simulink model "GTA_PCMFirmware"  (Simulink 7.8)
settings: Solver=FixedStepDiscrete  StartTime=0.0  StopTime=10.0  RelTol=1e-3
PreLoadFcn:
  | try, eval([bdroot '_setup']); catch, eval('model_setup', ''); end
InitFcn:
  | try, eval([bdroot '_setup']); catch, eval('model_setup', ''); end
undefined symbols (not defined in the file): fndFwd, fndNeut, fndRev, FWDlockout, GCM, keySwIgn2, motohawk_build_version, motohawk_trunc_name, motohawk_vardec_path, REVlockout
libraries: MotoHawk_lib x313, simulink x47, GTA_Library x13
(part 3 of 7)

== system GTA_PCMFirmware/Function/1 Inputs and Paramaters/Limits/Pb ==
  Mux : Mux  Inputs=13
  motohawk_calibration : MotoHawk_lib/Calibration & Probing Blocks/motohawk_calibration  nam='PbMaxCellVoltage'  val=PbMaxCellVoltage  storage=Calibration  show_more=off  name_source=Use Parameter  data_type=Inherit from 'Default Value'  read_level=1  write_level=1  ovr_cals=on  view_as=Number  enum_struct={'Disabled', 'Enabled'}  vector_style=Wide Row  use_help_units=off  help=''  units=''  use_header_enum=off  row_header_enum={}  col_header_enum={}  use_min_max=off  min_val=-inf  max_val=inf  use_precision=off  precision=''  gain=1  offset=0  exp=1  use_mototune_group=off  mototune_group=motohawk_vardec_path(gcb)
  motohawk_calibration1 : MotoHawk_lib/Calibration & Probing Blocks/motohawk_calibration  nam='PbMinCellVoltage'  val=PbMinCellVoltage  storage=Calibration  show_more=off  name_source=Use Parameter  data_type=Inherit from 'Default Value'  read_level=1  write_level=1  ovr_cals=on  view_as=Number  enum_struct={'Disabled', 'Enabled'}  vector_style=Wide Row  use_help_units=off  help=''  units=''  use_header_enum=off  row_header_enum={}  col_header_enum={}  use_min_max=off  min_val=-inf  max_val=inf  use_precision=off  precision=''  gain=1  offset=0  exp=1  use_mototune_group=off  mototune_group=motohawk_vardec_path(gcb)
  motohawk_calibration10 : MotoHawk_lib/Calibration & Probing Blocks/motohawk_calibration  nam='PbMotorCurrentScalar'  val=PbMotorCurrentScalar  storage=Calibration  show_more=off  name_source=Use Parameter  data_type=Inherit from 'Default Value'  read_level=1  write_level=1  ovr_cals=on  view_as=Number  enum_struct={'Disabled', 'Enabled'}  vector_style=Wide Row  use_help_units=off  help=''  units=''  use_header_enum=off  row_header_enum={}  col_header_enum={}  use_min_max=off  min_val=-inf  max_val=inf  use_precision=off  precision=''  gain=1  offset=0  exp=1  use_mototune_group=off  mototune_group=motohawk_vardec_path(gcb)
  motohawk_calibration11 : MotoHawk_lib/Calibration & Probing Blocks/motohawk_calibration  nam='PbMotorRegenScalar'  val=PbMotorRegenScalar  storage=Calibration  show_more=off  name_source=Use Parameter  data_type=Inherit from 'Default Value'  read_level=1  write_level=1  ovr_cals=on  view_as=Number  enum_struct={'Disabled', 'Enabled'}  vector_style=Wide Row  use_help_units=off  help=''  units=''  use_header_enum=off  row_header_enum={}  col_header_enum={}  use_min_max=off  min_val=-inf  max_val=inf  use_precision=off  precision=''  gain=1  offset=0  exp=1  use_mototune_group=off  mototune_group=motohawk_vardec_path(gcb)
  motohawk_calibration12 : MotoHawk_lib/Calibration & Probing Blocks/motohawk_calibration  nam='PbMaxRegenVoltage'  val=PbMaxRegenVoltage  storage=Calibration  show_more=off  name_source=Use Parameter  data_type=Inherit from 'Default Value'  read_level=1  write_level=1  ovr_cals=on  view_as=Number  enum_struct={'Disabled', 'Enabled'}  vector_style=Wide Row  use_help_units=off  help=''  units=''  use_header_enum=off  row_header_enum={}  col_header_enum={}  use_min_max=off  min_val=-inf  max_val=inf  use_precision=off  precision=''  gain=1  offset=0  exp=1  use_mototune_group=off  mototune_group=motohawk_vardec_path(gcb)
  motohawk_calibration2 : MotoHawk_lib/Calibration & Probing Blocks/motohawk_calibration  nam='PbCurrentLimit'  val=PbCurrentLimit  storage=Calibration  show_more=off  name_source=Use Parameter  data_type=Inherit from 'Default Value'  read_level=1  write_level=1  ovr_cals=on  view_as=Number  enum_struct={'Disabled', 'Enabled'}  vector_style=Wide Row  use_help_units=off  help=''  units=''  use_header_enum=off  row_header_enum={}  col_header_enum={}  use_min_max=off  min_val=-inf  max_val=inf  use_precision=off  precision=''  gain=1  offset=0  exp=1  use_mototune_group=off  mototune_group=motohawk_vardec_path(gcb)
  motohawk_calibration3 : MotoHawk_lib/Calibration & Probing Blocks/motohawk_calibration  nam='PbRegenLimit'  val=PbRegenLimit  storage=Calibration  show_more=off  name_source=Use Parameter  data_type=Inherit from 'Default Value'  read_level=1  write_level=1  ovr_cals=on  view_as=Number  enum_struct={'Disabled', 'Enabled'}  vector_style=Wide Row  use_help_units=off  help=''  units=''  use_header_enum=off  row_header_enum={}  col_header_enum={}  use_min_max=off  min_val=-inf  max_val=inf  use_precision=off  precision=''  gain=1  offset=0  exp=1  use_mototune_group=off  mototune_group=motohawk_vardec_path(gcb)
  motohawk_calibration4 : MotoHawk_lib/Calibration & Probing Blocks/motohawk_calibration  nam='PbMaxChargeTemp'  val=PbMaxChargeTemp  storage=Calibration  show_more=off  name_source=Use Parameter  data_type=Inherit from 'Default Value'  read_level=1  write_level=1  ovr_cals=on  view_as=Number  enum_struct={'Disabled', 'Enabled'}  vector_style=Wide Row  use_help_units=off  help=''  units=''  use_header_enum=off  row_header_enum={}  col_header_enum={}  use_min_max=off  min_val=-inf  max_val=inf  use_precision=off  precision=''  gain=1  offset=0  exp=1  use_mototune_group=off  mototune_group=motohawk_vardec_path(gcb)
  motohawk_calibration5 : MotoHawk_lib/Calibration & Probing Blocks/motohawk_calibration  nam='PbMinChargeTemp'  val=PbMinChargeTemp  storage=Calibration  show_more=off  name_source=Use Parameter  data_type=Inherit from 'Default Value'  read_level=1  write_level=1  ovr_cals=on  view_as=Number  enum_struct={'Disabled', 'Enabled'}  vector_style=Wide Row  use_help_units=off  help=''  units=''  use_header_enum=off  row_header_enum={}  col_header_enum={}  use_min_max=off  min_val=-inf  max_val=inf  use_precision=off  precision=''  gain=1  offset=0  exp=1  use_mototune_group=off  mototune_group=motohawk_vardec_path(gcb)
  motohawk_calibration6 : MotoHawk_lib/Calibration & Probing Blocks/motohawk_calibration  nam='PbMaxDischargeTemp'  val=PbMaxDischargeTemp  storage=Calibration  show_more=off  name_source=Use Parameter  data_type=Inherit from 'Default Value'  read_level=1  write_level=1  ovr_cals=on  view_as=Number  enum_struct={'Disabled', 'Enabled'}  vector_style=Wide Row  use_help_units=off  help=''  units=''  use_header_enum=off  row_header_enum={}  col_header_enum={}  use_min_max=off  min_val=-inf  max_val=inf  use_precision=off  precision=''  gain=1  offset=0  exp=1  use_mototune_group=off  mototune_group=motohawk_vardec_path(gcb)
  motohawk_calibration7 : MotoHawk_lib/Calibration & Probing Blocks/motohawk_calibration  nam='PbMinDischargeTemp'  val=PbMinDischargeTemp  storage=Calibration  show_more=off  name_source=Use Parameter  data_type=Inherit from 'Default Value'  read_level=1  write_level=1  ovr_cals=on  view_as=Number  enum_struct={'Disabled', 'Enabled'}  vector_style=Wide Row  use_help_units=off  help=''  units=''  use_header_enum=off  row_header_enum={}  col_header_enum={}  use_min_max=off  min_val=-inf  max_val=inf  use_precision=off  precision=''  gain=1  offset=0  exp=1  use_mototune_group=off  mototune_group=motohawk_vardec_path(gcb)
  motohawk_calibration8 : MotoHawk_lib/Calibration & Probing Blocks/motohawk_calibration  nam='PbMaxPackVoltage'  val=PbMaxPackVoltage  storage=Calibration  show_more=off  name_source=Use Parameter  data_type=Inherit from 'Default Value'  read_level=1  write_level=1  ovr_cals=on  view_as=Number  enum_struct={'Disabled', 'Enabled'}  vector_style=Wide Row  use_help_units=off  help=''  units=''  use_header_enum=off  row_header_enum={}  col_header_enum={}  use_min_max=off  min_val=-inf  max_val=inf  use_precision=off  precision=''  gain=1  offset=0  exp=1  use_mototune_group=off  mototune_group=motohawk_vardec_path(gcb)
  motohawk_calibration9 : MotoHawk_lib/Calibration & Probing Blocks/motohawk_calibration  nam='PbMinPackVoltage'  val=PbMinPackVoltage  storage=Calibration  show_more=off  name_source=Use Parameter  data_type=Inherit from 'Default Value'  read_level=1  write_level=1  ovr_cals=on  view_as=Number  enum_struct={'Disabled', 'Enabled'}  vector_style=Wide Row  use_help_units=off  help=''  units=''  use_header_enum=off  row_header_enum={}  col_header_enum={}  use_min_max=off  min_val=-inf  max_val=inf  use_precision=off  precision=''  gain=1  offset=0  exp=1  use_mototune_group=off  mototune_group=motohawk_vardec_path(gcb)
  PbPack : Outport
  wires:
  Mux/1 -> PbPack/1
  motohawk_calibration12/1 -> Mux/13  "MaxRegenVoltage"
  motohawk_calibration11/1 -> Mux/12  "MotorRegenScalar"
  motohawk_calibration10/1 -> Mux/11  "MotorCurrentScalar"
  motohawk_calibration9/1 -> Mux/10  "MinPackVoltage"
  motohawk_calibration8/1 -> Mux/9  "MaxPackVoltage"
  motohawk_calibration7/1 -> Mux/8  "MinDischargeTemp"
  motohawk_calibration6/1 -> Mux/7  "MaxDischargeTemp"
  motohawk_calibration5/1 -> Mux/6  "MinChargeTemp"
  motohawk_calibration4/1 -> Mux/5  "MaxChargeTemp"
  motohawk_calibration3/1 -> Mux/4  "RegenLimit"
  motohawk_calibration2/1 -> Mux/3  "CurrentLimit"
  motohawk_calibration1/1 -> Mux/2  "MinCellVoltage"
  motohawk_calibration/1 -> Mux/1  "MaxCellVoltage"

== system GTA_PCMFirmware/Function/2 Control Loop/Component Controls/Body Control ==
  SYSin : Inport
  MotorControl : Inport  Port=2
  Bus Creator : BusCreator  Inputs=3
  Defroster : Subsystem
  Inter Wiper : Subsystem
  Reverse Lights : Subsystem
  Out : Outport
  wires:
  SYSin/1 -> Defroster/1(SYSin), Inter Wiper/1(SYSin), Reverse Lights/1(SYSin)
  Inter Wiper/1(Out1) -> Bus Creator/2  "Wiper"
  Defroster/1(Out1) -> Bus Creator/1  "Defrost"
  Reverse Lights/1(Out1) -> Bus Creator/3  "ReverseLight"
  Bus Creator/1 -> Out/1
  MotorControl/1 -> Reverse Lights/2(MotorControl)

== system GTA_PCMFirmware/Function/2 Control Loop/Component Controls/Charger Control ==
  SYSin : Inport
  Bus Creator : BusCreator  Inputs=1
  Bus Selector : BusSelector  OutputSignals=ModeControl.ChargeEnable,BUS.Input Bus.CANin.BMS.csChargeFlags.PackCharging
  Logical Operator : Logic  AllPortsSameDT=off  OutDataTypeStr=boolean
  Out : Outport
  wires:
  SYSin/1 -> Bus Selector/1
  Bus Selector/1 -> Logical Operator/1  "<ChargeEnable>"
  Bus Selector/2 -> Logical Operator/2  "<PackCharging>"
  Logical Operator/1 -> Bus Creator/1  "ChargerOut"
  Bus Creator/1 -> Out/1

== system GTA_PCMFirmware/Function/2 Control Loop/Component Controls/Display Control ==
  SYSin : Inport
  MotorControl : Inport  Port=2
  Bus Creator : BusCreator
  Fault Lamps : Subsystem
  Gearbox Display : Subsystem
  ReadyLight : Subsystem
  Vehicle Speed : Subsystem
  Out : Outport
  wires:
  SYSin/1 -> Fault Lamps/1(SYSin), Gearbox Display/1(SYSin), Vehicle Speed/1(SYSin), ReadyLight/1(SYSin)
  Fault Lamps/1(FaultLights) -> Bus Creator/1  "FaultLamp"
  Vehicle Speed/1(Out1) -> Bus Creator/3  "VehSpeed"
  Gearbox Display/1(GboxPos) -> Bus Creator/2  "GearDisp"
  Bus Creator/1 -> Out/1
  ReadyLight/1(ReadyLight) -> Bus Creator/4  "ReadyLight"
  MotorControl/1 -> Gearbox Display/2(MotorControl)

== system GTA_PCMFirmware/Function/2 Control Loop/Component Controls/Motor Control ==
  SYSin : Inport
  Bus Creator : BusCreator  Inputs=3
  Bus Selector : BusSelector  OutputSignals=ModeControl.DriveEnable,BUS.Input Bus.CANin.Motor Controller.KinVoltSpeed.ErrorField
  Bus Selector1 : BusSelector  OutputSignals=BUS.Input Bus.DigitalIn.Shifter.ShifterPos,BUS.Input Bus.CANin.Motor Controller.KinVoltSpeed.MotorSpeed,BUS.Input Bus.CANin.Motor Controller.KinCurrFB.iq_ref
  Bus Selector2 : BusSelector  OutputSignals=ModeControl.MotorEnable,BUS.Input Bus.DigitalIn.Shifter.ShifterPos,BUS.Input Bus.DigitalIn.KeySwitch.KeySw,BUS.Input Bus.AnalogIn.ThrottlePedal.PedalPerc,BUS.Input Bus.CANin.Motor Controller.KinVoltSpeed.MotorSpeed,BUS.Current Limit.TorqueLimit.MaxCurrPerc,BUS.Current Limit.RegenLimit.MaxRegenPerc,BUS.Input Bus.Limits.BattLimits.MotorRegenScalar,BUS.Input Bus.Limits.BattLimits.MotorCurrentScalar
  Current Request Algorithm : Subsystem
  Direction Lockout : Subsystem
  Direction Selector & Control Loop : Subsystem
  Enable : Subsystem
  Out : Outport
  wires:
  Enable/1(enable) -> Bus Creator/1
  Direction Lockout/1(" FNDOut") -> Direction Selector & Control Loop/1(" FNDSw"), Current Request Algorithm/4(FNDOut), Bus Creator/2
  Bus Selector1/1 -> Direction Lockout/1(" FNDSw")  "<ShifterPos>"
  Bus Selector1/2 -> Direction Selector & Control Loop/4(Speed), Direction Lockout/2(" Speed")  "<MotorSpeed>"
  Current Request Algorithm/1(torqueRequest) -> Direction Selector & Control Loop/2(" torque")
  Direction Selector & Control Loop/1(torqueOutput) -> Bus Creator/3
  Bus Selector1/3 -> Direction Selector & Control Loop/3(CurFBK)  "<iq_ref>"
  Bus Selector/1 -> Enable/1("driveEnable ")  "<DriveEnable>"
  Bus Selector/2 -> Enable/2(errorField)  "<ErrorField>"
  SYSin/1 -> Bus Selector1/1, Bus Selector/1, Bus Selector2/1
  Bus Selector2/1 -> Current Request Algorithm/1(MotorEnable)  "<MotorEnable>"
  Bus Selector2/2 -> Current Request Algorithm/2("FNDSwitch ")  "<ShifterPos>"
  Bus Selector2/3 -> Current Request Algorithm/3(KeySwitch)  "<KeySw>"
  Bus Selector2/4 -> Current Request Algorithm/5("Pedal ")  "<PedalPerc>"
  Bus Selector2/5 -> Current Request Algorithm/6(Speed)  "<MotorSpeed>"
  Bus Selector2/6 -> Current Request Algorithm/7("TorqueLim ")  "<MaxCurrPerc>"
  Bus Selector2/7 -> Current Request Algorithm/8(RegenLim)  "<MaxRegenPerc>"
  Bus Selector2/8 -> Current Request Algorithm/9(RegenScalar)  "<MotorRegenScalar>"
  Bus Selector2/9 -> Current Request Algorithm/10(CurrentScalar)  "<MotorCurrentScalar>"
  Bus Creator/1 -> Out/1

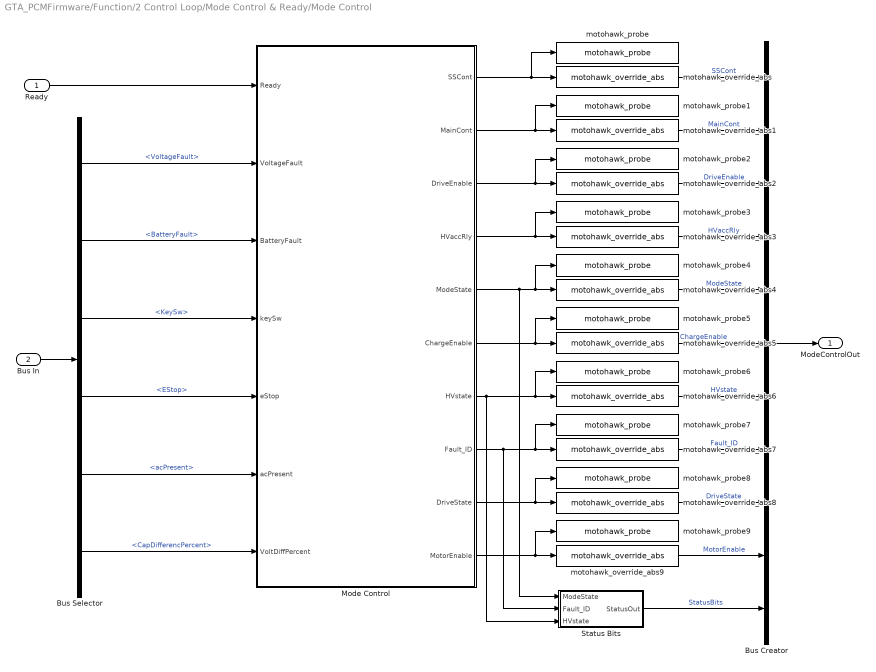
== system GTA_PCMFirmware/Function/2 Control Loop/Mode Control & Ready/Mode Control ==
  Ready : Inport
  Bus In : Inport  Port=2
  Bus Creator : BusCreator  Inputs=11
  Bus Selector : BusSelector  OutputSignals=Voltage level.VoltageFault,Faults.BatteryFault.BatteryFault,Input Bus.DigitalIn.KeySwitch.KeySw,Input Bus.DigitalIn.EStop.EStop,Input Bus.DigitalIn.Charger.acPresent,Voltage level.CapDifferencPercent
  Mode Control : Stateflow chart  TreatAsAtomicUnit=on
  Status Bits : Subsystem
  motohawk_override_abs : MotoHawk_lib/Calibration & Probing Blocks/motohawk_override_abs  parent_name='SScont'  parent_val=0  show_more=off  name_source=Use Parameter  parent_read_level=1  parent_override_level=1  view_as=Number  enum_struct={'Disabled', 'Enabled'}  use_help_units=off  parent_help=''  parent_units=''  use_min_max=off  parent_min=-inf  parent_max=inf  use_precision=off  parent_precision=''  parent_gain=1  parent_offset=0  parent_exp=1  use_mototune_group=off  parent_group=motohawk_vardec_path(gcb)
  motohawk_override_abs1 : MotoHawk_lib/Calibration & Probing Blocks/motohawk_override_abs  parent_name='MainCont'  parent_val=0  show_more=off  name_source=Use Parameter  parent_read_level=1  parent_override_level=1  view_as=Number  enum_struct={'Disabled', 'Enabled'}  use_help_units=off  parent_help=''  parent_units=''  use_min_max=off  parent_min=-inf  parent_max=inf  use_precision=off  parent_precision=''  parent_gain=1  parent_offset=0  parent_exp=1  use_mototune_group=off  parent_group=motohawk_vardec_path(gcb)
  motohawk_override_abs2 : MotoHawk_lib/Calibration & Probing Blocks/motohawk_override_abs  parent_name='DriveEnable'  parent_val=0  show_more=off  name_source=Use Parameter  parent_read_level=1  parent_override_level=1  view_as=Number  enum_struct={'Disabled', 'Enabled'}  use_help_units=off  parent_help=''  parent_units=''  use_min_max=off  parent_min=-inf  parent_max=inf  use_precision=off  parent_precision=''  parent_gain=1  parent_offset=0  parent_exp=1  use_mototune_group=off  parent_group=motohawk_vardec_path(gcb)
  motohawk_override_abs3 : MotoHawk_lib/Calibration & Probing Blocks/motohawk_override_abs  parent_name='HVaccRly'  parent_val=0  show_more=off  name_source=Use Parameter  parent_read_level=1  parent_override_level=1  view_as=Number  enum_struct={'Disabled', 'Enabled'}  use_help_units=off  parent_help=''  parent_units=''  use_min_max=off  parent_min=-inf  parent_max=inf  use_precision=off  parent_precision=''  parent_gain=1  parent_offset=0  parent_exp=1  use_mototune_group=off  parent_group=motohawk_vardec_path(gcb)
  motohawk_override_abs4 : MotoHawk_lib/Calibration & Probing Blocks/motohawk_override_abs  parent_name='ModeState'  parent_val=0  show_more=off  name_source=Use Parameter  parent_read_level=1  parent_override_level=1  view_as=Number  enum_struct={'Disabled', 'Enabled'}  use_help_units=off  parent_help=''  parent_units=''  use_min_max=off  parent_min=-inf  parent_max=inf  use_precision=off  parent_precision=''  parent_gain=1  parent_offset=0  parent_exp=1  use_mototune_group=off  parent_group=motohawk_vardec_path(gcb)
  motohawk_override_abs5 : MotoHawk_lib/Calibration & Probing Blocks/motohawk_override_abs  parent_name='ChargeEnable'  parent_val=0  show_more=off  name_source=Use Parameter  parent_read_level=1  parent_override_level=1  view_as=Number  enum_struct={'Disabled', 'Enabled'}  use_help_units=off  parent_help=''  parent_units=''  use_min_max=off  parent_min=-inf  parent_max=inf  use_precision=off  parent_precision=''  parent_gain=1  parent_offset=0  parent_exp=1  use_mototune_group=off  parent_group=motohawk_vardec_path(gcb)
  motohawk_override_abs6 : MotoHawk_lib/Calibration & Probing Blocks/motohawk_override_abs  parent_name='HVstate'  parent_val=0  show_more=off  name_source=Use Parameter  parent_read_level=1  parent_override_level=1  view_as=Number  enum_struct={'Disabled', 'Enabled'}  use_help_units=off  parent_help=''  parent_units=''  use_min_max=off  parent_min=-inf  parent_max=inf  use_precision=off  parent_precision=''  parent_gain=1  parent_offset=0  parent_exp=1  use_mototune_group=off  parent_group=motohawk_vardec_path(gcb)
  motohawk_override_abs7 : MotoHawk_lib/Calibration & Probing Blocks/motohawk_override_abs  parent_name='Fault_ID'  parent_val=0  show_more=off  name_source=Use Parameter  parent_read_level=1  parent_override_level=1  view_as=Number  enum_struct={'Disabled', 'Enabled'}  use_help_units=off  parent_help=''  parent_units=''  use_min_max=off  parent_min=-inf  parent_max=inf  use_precision=off  parent_precision=''  parent_gain=1  parent_offset=0  parent_exp=1  use_mototune_group=off  parent_group=motohawk_vardec_path(gcb)
  motohawk_override_abs8 : MotoHawk_lib/Calibration & Probing Blocks/motohawk_override_abs  parent_name='DriveState'  parent_val=0  show_more=off  name_source=Use Parameter  parent_read_level=1  parent_override_level=1  view_as=Number  enum_struct={'Disabled', 'Enabled'}  use_help_units=off  parent_help=''  parent_units=''  use_min_max=off  parent_min=-inf  parent_max=inf  use_precision=off  parent_precision=''  parent_gain=1  parent_offset=0  parent_exp=1  use_mototune_group=off  parent_group=motohawk_vardec_path(gcb)
  motohawk_override_abs9 : MotoHawk_lib/Calibration & Probing Blocks/motohawk_override_abs  parent_name='MotorEnable'  parent_val=0  show_more=off  name_source=Use Parameter  parent_read_level=1  parent_override_level=1  view_as=Number  enum_struct={'Disabled', 'Enabled'}  use_help_units=off  parent_help=''  parent_units=''  use_min_max=off  parent_min=-inf  parent_max=inf  use_precision=off  parent_precision=''  parent_gain=1  parent_offset=0  parent_exp=1  use_mototune_group=off  parent_group=motohawk_vardec_path(gcb)
  motohawk_probe : MotoHawk_lib/Calibration & Probing Blocks/motohawk_probe  nam='SScont'  show_more=off  name_source=Use Parameter  read_level=1  view_as=Number  enum_struct={'Disabled', 'Enabled'}  vector_style=Wide Row  use_help_units=off  help=''  units=''  use_header_enum=off  row_header_enum={}  col_header_enum={}  use_min_max=off  min_val=-inf  max_val=inf  use_precision=off  precision=''  gain=1  offset=0  exp=1  use_mototune_group=off  mototune_group=motohawk_vardec_path(gcb)
  motohawk_probe1 : MotoHawk_lib/Calibration & Probing Blocks/motohawk_probe  nam='MainCont'  show_more=off  name_source=Use Parameter  read_level=1  view_as=Number  enum_struct={'Disabled', 'Enabled'}  vector_style=Wide Row  use_help_units=off  help=''  units=''  use_header_enum=off  row_header_enum={}  col_header_enum={}  use_min_max=off  min_val=-inf  max_val=inf  use_precision=off  precision=''  gain=1  offset=0  exp=1  use_mototune_group=off  mototune_group=motohawk_vardec_path(gcb)
  motohawk_probe2 : MotoHawk_lib/Calibration & Probing Blocks/motohawk_probe  nam='DriveEnable'  show_more=off  name_source=Use Parameter  read_level=1  view_as=Number  enum_struct={'Disabled', 'Enabled'}  vector_style=Wide Row  use_help_units=off  help=''  units=''  use_header_enum=off  row_header_enum={}  col_header_enum={}  use_min_max=off  min_val=-inf  max_val=inf  use_precision=off  precision=''  gain=1  offset=0  exp=1  use_mototune_group=off  mototune_group=motohawk_vardec_path(gcb)
  motohawk_probe3 : MotoHawk_lib/Calibration & Probing Blocks/motohawk_probe  nam='HVaccRly'  show_more=off  name_source=Use Parameter  read_level=1  view_as=Number  enum_struct={'Disabled', 'Enabled'}  vector_style=Wide Row  use_help_units=off  help=''  units=''  use_header_enum=off  row_header_enum={}  col_header_enum={}  use_min_max=off  min_val=-inf  max_val=inf  use_precision=off  precision=''  gain=1  offset=0  exp=1  use_mototune_group=off  mototune_group=motohawk_vardec_path(gcb)
  motohawk_probe4 : MotoHawk_lib/Calibration & Probing Blocks/motohawk_probe  nam='ModeState'  show_more=off  name_source=Use Parameter  read_level=1  view_as=Number  enum_struct={'Disabled', 'Enabled'}  vector_style=Wide Row  use_help_units=off  help=''  units=''  use_header_enum=off  row_header_enum={}  col_header_enum={}  use_min_max=off  min_val=-inf  max_val=inf  use_precision=off  precision=''  gain=1  offset=0  exp=1  use_mototune_group=off  mototune_group=motohawk_vardec_path(gcb)
  motohawk_probe5 : MotoHawk_lib/Calibration & Probing Blocks/motohawk_probe  nam='ChargeEnable'  show_more=off  name_source=Use Parameter  read_level=1  view_as=Number  enum_struct={'Disabled', 'Enabled'}  vector_style=Wide Row  use_help_units=off  help=''  units=''  use_header_enum=off  row_header_enum={}  col_header_enum={}  use_min_max=off  min_val=-inf  max_val=inf  use_precision=off  precision=''  gain=1  offset=0  exp=1  use_mototune_group=off  mototune_group=motohawk_vardec_path(gcb)
  motohawk_probe6 : MotoHawk_lib/Calibration & Probing Blocks/motohawk_probe  nam='HVstate'  show_more=off  name_source=Use Parameter  read_level=1  view_as=Number  enum_struct={'Disabled', 'Enabled'}  vector_style=Wide Row  use_help_units=off  help=''  units=''  use_header_enum=off  row_header_enum={}  col_header_enum={}  use_min_max=off  min_val=-inf  max_val=inf  use_precision=off  precision=''  gain=1  offset=0  exp=1  use_mototune_group=off  mototune_group=motohawk_vardec_path(gcb)
  motohawk_probe7 : MotoHawk_lib/Calibration & Probing Blocks/motohawk_probe  nam='Fault_ID'  show_more=off  name_source=Use Parameter  read_level=1  view_as=Number  enum_struct={'Disabled', 'Enabled'}  vector_style=Wide Row  use_help_units=off  help=''  units=''  use_header_enum=off  row_header_enum={}  col_header_enum={}  use_min_max=off  min_val=-inf  max_val=inf  use_precision=off  precision=''  gain=1  offset=0  exp=1  use_mototune_group=off  mototune_group=motohawk_vardec_path(gcb)
  motohawk_probe8 : MotoHawk_lib/Calibration & Probing Blocks/motohawk_probe  nam='DriveState'  show_more=off  name_source=Use Parameter  read_level=1  view_as=Number  enum_struct={'Disabled', 'Enabled'}  vector_style=Wide Row  use_help_units=off  help=''  units=''  use_header_enum=off  row_header_enum={}  col_header_enum={}  use_min_max=off  min_val=-inf  max_val=inf  use_precision=off  precision=''  gain=1  offset=0  exp=1  use_mototune_group=off  mototune_group=motohawk_vardec_path(gcb)
  motohawk_probe9 : MotoHawk_lib/Calibration & Probing Blocks/motohawk_probe  nam='MotorEnable'  show_more=off  name_source=Use Parameter  read_level=1  view_as=Number  enum_struct={'Disabled', 'Enabled'}  vector_style=Wide Row  use_help_units=off  help=''  units=''  use_header_enum=off  row_header_enum={}  col_header_enum={}  use_min_max=off  min_val=-inf  max_val=inf  use_precision=off  precision=''  gain=1  offset=0  exp=1  use_mototune_group=off  mototune_group=motohawk_vardec_path(gcb)
  ModeControlOut : Outport
  wires:
  Ready/1 -> Mode Control/1(Ready)
  Bus Creator/1 -> ModeControlOut/1
  Mode Control/1(SSCont) -> motohawk_override_abs/1, motohawk_probe/1
  Mode Control/2(MainCont) -> motohawk_override_abs1/1, motohawk_probe1/1
  Mode Control/3(DriveEnable) -> motohawk_override_abs2/1, motohawk_probe2/1
  Mode Control/4(HVaccRly) -> motohawk_override_abs3/1, motohawk_probe3/1
  Mode Control/5(ModeState) -> motohawk_override_abs4/1, motohawk_probe4/1, Status Bits/1(ModeState)
  Mode Control/6(ChargeEnable) -> motohawk_override_abs5/1, motohawk_probe5/1
  Mode Control/7(HVstate) -> motohawk_override_abs6/1, motohawk_probe6/1, Status Bits/3(HVstate)
  Mode Control/8(Fault_ID) -> motohawk_override_abs7/1, motohawk_probe7/1, Status Bits/2(Fault_ID)
  Mode Control/9(DriveState) -> motohawk_override_abs8/1, motohawk_probe8/1
  Mode Control/10(MotorEnable) -> motohawk_override_abs9/1, motohawk_probe9/1
  motohawk_override_abs9/1 -> Bus Creator/10  "MotorEnable"
  motohawk_override_abs8/1 -> Bus Creator/9  "DriveState"
  motohawk_override_abs7/1 -> Bus Creator/8  "Fault_ID"
  motohawk_override_abs6/1 -> Bus Creator/7  "HVstate"
  motohawk_override_abs5/1 -> Bus Creator/6  "ChargeEnable"
  motohawk_override_abs4/1 -> Bus Creator/5  "ModeState"
  motohawk_override_abs3/1 -> Bus Creator/4  "HVaccRly"
  motohawk_override_abs2/1 -> Bus Creator/3  "DriveEnable"
  motohawk_override_abs1/1 -> Bus Creator/2  "MainCont"
  motohawk_override_abs/1 -> Bus Creator/1  "SSCont"
  Bus In/1 -> Bus Selector/1
  Bus Selector/4 -> Mode Control/5(eStop)  "<EStop>"
  Bus Selector/5 -> Mode Control/6(acPresent)  "<acPresent>"
  Bus Selector/1 -> Mode Control/2(VoltageFault)  "<VoltageFault>"
  Bus Selector/6 -> Mode Control/7(VoltDiffPercent)  "<CapDifferencPercent>"
  Bus Selector/3 -> Mode Control/4(keySw)  "<KeySw>"
  Bus Selector/2 -> Mode Control/3(BatteryFault)  "<BatteryFault>"
  Status Bits/1(StatusOut) -> Bus Creator/11  "StatusBits"

== system GTA_PCMFirmware/Function/2 Control Loop/Mode Control & Ready/Ready ==
  Inputs : Inport
  Bitwise Operator : simulink/Logic and Bit Operations/Bitwise Operator  logicop=AND  UseBitMask=on  BitMask=keySwIgn2  BitMaskRealWorld=Stored Integer
  Bus Selector : BusSelector  OutputSignals=Input Bus.DigitalIn.Shifter.ShifterPos,Input Bus.DigitalIn.Shifter.dbgShifter.sbgShiftErr,Input Bus.DigitalIn.KeySwitch.KeySw,Input Bus.DigitalIn.EStop.EStop,Input Bus.DigitalIn.Charger.acPresent
  Compare To Constant : simulink/Logic and Bit Operations/Compare To Constant  relop===  const=fndNeut  OutDataTypeStr=boolean
  Logical Operator : Logic  Operator=NOT  AllPortsSameDT=off  OutDataTypeStr=boolean
  Logical Operator1 : Logic  Operator=OR  Inputs=1  AllPortsSameDT=off  OutDataTypeStr=boolean
  Logical Operator2 : Logic  Operator=NOT  AllPortsSameDT=off  OutDataTypeStr=boolean
  Logical Operator3 : Logic  Operator=NOT  AllPortsSameDT=off  OutDataTypeStr=boolean
  Logical Operator4 : Logic  Inputs=1  AllPortsSameDT=off  OutDataTypeStr=boolean
  Mux : Mux  Inputs=5
  motohawk_probe : MotoHawk_lib/Calibration & Probing Blocks/motohawk_probe  nam='ReadyState'  show_more=off  name_source=Use Parameter  read_level=1  view_as=Number  enum_struct={'Disabled', 'Enabled'}  vector_style=Wide Row  use_help_units=off  help=''  units=''  use_header_enum=off  row_header_enum={}  col_header_enum={}  use_min_max=off  min_val=-inf  max_val=inf  use_precision=off  precision=''  gain=1  offset=0  exp=1  use_mototune_group=off  mototune_group=motohawk_vardec_path(gcb)
  Ready : Outport
  wires:
  Inputs/1 -> Bus Selector/1
  Bus Selector/1 -> Compare To Constant/1  "<ShifterPos>"
  Bus Selector/2 -> Logical Operator/1  "<sbgShiftErr>"
  Bus Selector/3 -> Bitwise Operator/1  "<KeySw>"
  Bitwise Operator/1 -> Logical Operator1/1
  Bus Selector/4 -> Logical Operator2/1  "<EStop>"
  Bus Selector/5 -> Logical Operator3/1  "<acPresent>"
  Compare To Constant/1 -> Mux/1
  Logical Operator3/1 -> Mux/5
  Logical Operator2/1 -> Mux/4
  Logical Operator1/1 -> Mux/3
  Logical Operator/1 -> Mux/2
  Logical Operator4/1 -> Ready/1
  Mux/1 -> Logical Operator4/1, motohawk_probe/1

== system GTA_PCMFirmware/Function/2 Control Loop/Safety/Current Limit ==
  Input Bus : Inport
  Bus Creator : BusCreator  Inputs=2
  RegenLimit : Subsystem
  TorqueLimit : Subsystem
  CurrentLimits : Outport
  wires:
  Input Bus/1 -> TorqueLimit/1(InputBus), RegenLimit/1(InputBus)
  TorqueLimit/1(Out) -> Bus Creator/1  "TorqueLimit"
  RegenLimit/1(Out) -> Bus Creator/2  "RegenLimit"
  Bus Creator/1 -> CurrentLimits/1

== system GTA_PCMFirmware/Function/2 Control Loop/Safety/Faults ==
  Input Bus : Inport
  BatteryFault : Subsystem
  Bus Creator : BusCreator  Inputs=1
  Out1 : Outport
  wires:
  Bus Creator/1 -> Out1/1
  Input Bus/1 -> BatteryFault/1(InputBus)
  BatteryFault/1(BatteryFault) -> Bus Creator/1  "BatteryFault"

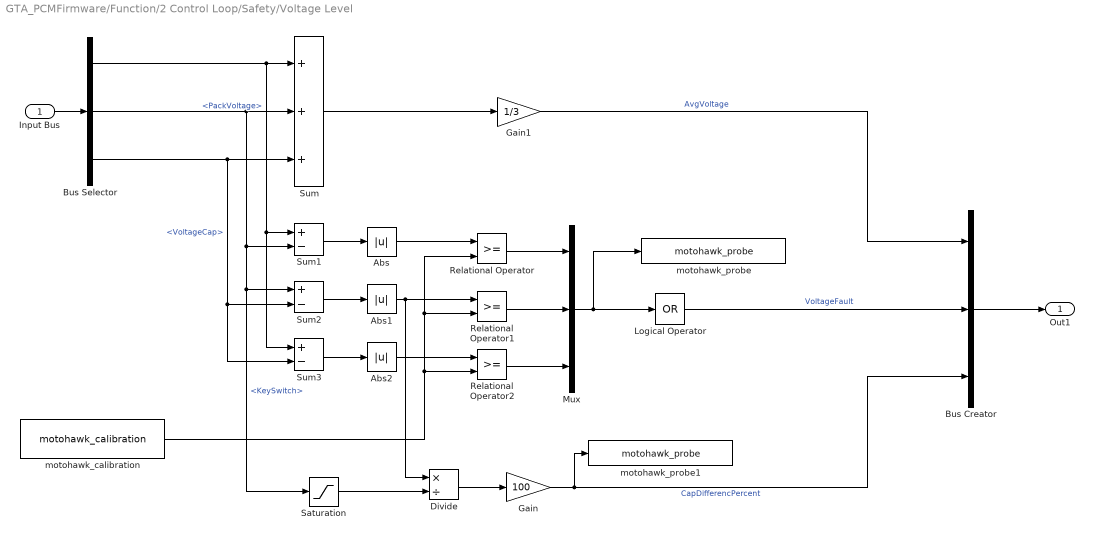
== system GTA_PCMFirmware/Function/2 Control Loop/Safety/Voltage Level ==
  Input Bus : Inport
  Abs : Abs
  Abs1 : Abs
  Abs2 : Abs
  Bus Creator : BusCreator  Inputs=3
  Bus Selector : BusSelector  OutputSignals=CANin.BMS.csCellInfo.PackVoltage,CANin.Motor Controller.KinVoltSpeed.KeySwitch,CANin.Motor Controller.KinVoltSpeed.VoltageCap
  Divide : Product  Inputs=*/
  Gain : Gain  Gain=100
  Gain1 : Gain  Gain=1/3
  Logical Operator : Logic  Operator=OR  Inputs=1  AllPortsSameDT=off  OutDataTypeStr=boolean
  Mux : Mux  Inputs=3
  Relational Operator : RelationalOperator  OutDataTypeStr=boolean
  Relational Operator1 : RelationalOperator  OutDataTypeStr=boolean
  Relational Operator2 : RelationalOperator  OutDataTypeStr=boolean
  Saturation : Saturate  UpperLimit=150  LowerLimit=5
  Sum : Sum  Inputs=+++
  Sum1 : Sum  Inputs=+-
  Sum2 : Sum  Inputs=+-
  Sum3 : Sum  Inputs=+-
  motohawk_calibration : MotoHawk_lib/Calibration & Probing Blocks/motohawk_calibration  nam='AllowableVoltageDelta'  val=AllowableVoltageDelta  storage=Calibration  show_more=off  name_source=Use Parameter  data_type=Inherit from 'Default Value'  read_level=1  write_level=1  ovr_cals=on  view_as=Number  enum_struct={'Disabled', 'Enabled'}  vector_style=Wide Row  use_help_units=off  help=''  units=''  use_header_enum=off  row_header_enum={}  col_header_enum={}  use_min_max=off  min_val=-inf  max_val=inf  use_precision=off  precision=''  gain=1  offset=0  exp=1  use_mototune_group=off  mototune_group=motohawk_vardec_path(gcb)
  motohawk_probe : MotoHawk_lib/Calibration & Probing Blocks/motohawk_probe  nam='VoltageFaults'  show_more=off  name_source=Use Parameter  read_level=1  view_as=Number  enum_struct={'Disabled', 'Enabled'}  vector_style=Wide Row  use_help_units=off  help=''  units=''  use_header_enum=off  row_header_enum={}  col_header_enum={}  use_min_max=off  min_val=-inf  max_val=inf  use_precision=off  precision=''  gain=1  offset=0  exp=1  use_mototune_group=off  mototune_group=motohawk_vardec_path(gcb)
  motohawk_probe1 : MotoHawk_lib/Calibration & Probing Blocks/motohawk_probe  nam='VoltDiffPercent'  show_more=off  name_source=Use Parameter  read_level=1  view_as=Number  enum_struct={'Disabled', 'Enabled'}  vector_style=Wide Row  use_help_units=off  help=''  units=''  use_header_enum=off  row_header_enum={}  col_header_enum={}  use_min_max=off  min_val=-inf  max_val=inf  use_precision=off  precision=''  gain=1  offset=0  exp=1  use_mototune_group=off  mototune_group=motohawk_vardec_path(gcb)
  Out1 : Outport
  wires:
  Input Bus/1 -> Bus Selector/1
  Bus Selector/2 -> Sum/2, Sum1/2, Sum2/1, Saturation/1  "<KeySwitch>"
  Bus Selector/1 -> Sum/1, Sum1/1, Sum3/1  "<PackVoltage>"
  Bus Selector/3 -> Sum/3, Sum2/2, Sum3/2  "<VoltageCap>"
  Sum1/1 -> Abs/1
  Sum2/1 -> Abs1/1
  Sum3/1 -> Abs2/1
  Abs/1 -> Relational Operator/1
  motohawk_calibration/1 -> Relational Operator/2, Relational Operator1/2, Relational Operator2/2
  Abs1/1 -> Relational Operator1/1, Divide/1
  Abs2/1 -> Relational Operator2/1
  Divide/1 -> Gain/1
  Relational Operator1/1 -> Mux/2
  Relational Operator2/1 -> Mux/3
  Relational Operator/1 -> Mux/1
  Mux/1 -> Logical Operator/1, motohawk_probe/1
  Sum/1 -> Gain1/1
  Gain1/1 -> Bus Creator/1  "AvgVoltage"
  Logical Operator/1 -> Bus Creator/2  "VoltageFault"
  Gain/1 -> motohawk_probe1/1, Bus Creator/3  "CapDifferencPercent"
  Bus Creator/1 -> Out1/1
  Saturation/1 -> Divide/2

== system GTA_PCMFirmware/Function/3 Output and Debug/CAN/Charger ==
  null : Inport
  Terminator1 : Terminator
  wires:
  null/1 -> Terminator1/1

== system GTA_PCMFirmware/Function/3 Output and Debug/CAN/Current Sensor ==
  null : Inport
  Constant : Constant  Value=162  OutDataTypeStr=uint8
  Constant1 : Constant  Value=251  OutDataTypeStr=uint8
  Send CAN Messages : MotoHawk_lib/CAN Blocks/Send CAN Messages  bus=-2  nam='BMS_CAN'  msgl=CANMSG_FluxPowerCSQuery  pace=5  labelwires=off
  Terminator1 : Terminator
  wires:
  null/1 -> Terminator1/1
  Constant1/1 -> Send CAN Messages/2
  Constant/1 -> Send CAN Messages/1

== system GTA_PCMFirmware/Function/3 Output and Debug/CAN/Debug ==
  Debug In : Inport
  Message 0x700 : Subsystem
  Message 0x701 : Subsystem
  Message 0x702 : Subsystem
  Message 0x703 : Subsystem
  Message 0x704 : Subsystem
  wires:
  Debug In/1 -> Message 0x700/1(In1), Message 0x701/1(In1), Message 0x703/1(In1), Message 0x704/1(In1), Message 0x702/1(In1)

== system GTA_PCMFirmware/Function/3 Output and Debug/CAN/Instrument Cluster ==
  InputBus : Inport
  ControlBus : Inport  Port=2
  MCU : Subsystem
  VMS : Subsystem
  wires:
  ControlBus/1 -> VMS/2(ControlBus)
  InputBus/1 -> MCU/1(InputBus), VMS/1(InputBus)

== system GTA_PCMFirmware/Function/3 Output and Debug/CAN/MotorController ==
  InputBus : Inport
  ControlBus : Inport  Port=2
  Controller Command : Subsystem
  Watchdog : Subsystem
  wires:
  ControlBus/1 -> Controller Command/1(In1)
  InputBus/1 -> Watchdog/1(In1)

== system GTA_PCMFirmware/Function/3 Output and Debug/Debug Logic/IGN1 Logic ==
  InputBus : Inport
  Bus Selector : BusSelector  OutputSignals=DigitalIn.Charger.acPresent,DigitalIn.KeySwitch.KeySw
  Compare To Constant : simulink/Logic and Bit Operations/Compare To Constant  relop=>=  const=1  OutDataTypeStr=uint8
  Logical Operator : Logic  Operator=OR  AllPortsSameDT=off  OutDataTypeStr=boolean
  NOT : Logic  Operator=NOT  AllPortsSameDT=off  OutDataTypeStr=boolean
  Ign1 : Outport
  wires:
  Bus Selector/1 -> NOT/1  "<acPresent>"
  Bus Selector/2 -> Compare To Constant/1  "<KeySw>"
  Compare To Constant/1 -> Logical Operator/2
  NOT/1 -> Logical Operator/1
  Logical Operator/1 -> Ign1/1  "IGN1"
  InputBus/1 -> Bus Selector/1

== system GTA_PCMFirmware/Function/3 Output and Debug/Debug Logic/InverterOT ==
  InputBus : Inport
  Bus Selector : BusSelector  OutputSignals=CANin.Motor Controller.KinTempWarn.HeatSinkTemp,SysParams.invOverTemp
  Relational Operator : RelationalOperator  OutDataTypeStr=boolean
  InverterOT : Outport
  wires:
  Bus Selector/1 -> Relational Operator/1  "<HeatSinkTemp>"
  Relational Operator/1 -> InverterOT/1
  InputBus/1 -> Bus Selector/1
  Bus Selector/2 -> Relational Operator/2  "<invOverTemp>"

== system GTA_PCMFirmware/Function/3 Output and Debug/Debug Logic/MotorOT ==
  InputBus : Inport
  Bus Selector : BusSelector  OutputSignals=CANin.Motor Controller.KinTempWarn.MotorTemp,SysParams.motorOverTemp
  Relational Operator : RelationalOperator  Operator=<=  OutDataTypeStr=boolean
  MotorOT : Outport
  wires:
  InputBus/1 -> Bus Selector/1
  Bus Selector/1 -> Relational Operator/1  "<MotorTemp>"
  Bus Selector/2 -> Relational Operator/2  "<motorOverTemp>"
  Relational Operator/1 -> MotorOT/1

== system GTA_PCMFirmware/Function/3 Output and Debug/Debug Logic/SOCok ==
  InputBus : Inport
  Bus Selector : BusSelector  OutputSignals=CANin.BMS.csInfo.UserSOC
  Compare To Constant : simulink/Logic and Bit Operations/Compare To Constant  relop=>  const=0  OutDataTypeStr=boolean
  SOCok : Outport
  wires:
  InputBus/1 -> Bus Selector/1
  Compare To Constant/1 -> SOCok/1
  Bus Selector/1 -> Compare To Constant/1  "<UserSOC>"

== system GTA_PCMFirmware/Function/1 Inputs and Paramaters/Analog/Throttle Pedal/FilterAndNormalize ==
  In1 : Inport
  Data Type Conversion : DataTypeConversion  OutDataTypeStr=single
  Discrete FIR Filter : DiscreteFir  Coefficients=ones(1,10)/10
  Out1 : Outport
  wires:
  In1/1 -> Data Type Conversion/1
  Data Type Conversion/1 -> Discrete FIR Filter/1
  Discrete FIR Filter/1 -> Out1/1

== system GTA_PCMFirmware/Function/1 Inputs and Paramaters/Analog/Throttle Pedal/ThrottlePedal ==
  Pedal1 : Inport
  Supply : Inport  Port=2
  Pedal2 : Inport  Port=3
  Divide : Product  Inputs=*/
  Divide1 : Product  Inputs=/*
  Gain : Gain  Gain=100
  Gain1 : Gain  Gain=100
  Gain2 : Gain  Gain=2
  Gain3 : Gain  Gain=2
  Interval Test : simulink/Logic and Bit Operations/Interval Test  IntervalClosedRight=on  uplimit=45  IntervalClosedLeft=on  lowlimit=7  OutDataTypeStr=uint8
  Interval Test1 : simulink/Logic and Bit Operations/Interval Test  IntervalClosedRight=on  uplimit=90  IntervalClosedLeft=on  lowlimit=15  OutDataTypeStr=uint8
  Logical Operator : Logic  Operator=OR  AllPortsSameDT=off  OutDataTypeStr=boolean
  Pot->% : Lookup_n-D  NumberOfTableDimensions=1  BreakpointsForDimension1=[20 84]  Table=[0 100]  ExtrapMethod=Clip  UseLastTableValue=on  OutDataTypeStr=single  RndMeth=Simplest  InputSameDT=on
  Product : Product  Inputs=3  RndMeth=Zero
  Relational Operator : RelationalOperator  Operator=<=  OutDataTypeStr=fixdt(0,8)
  Switch : Switch
  motohawk_probe : MotoHawk_lib/Calibration & Probing Blocks/motohawk_probe  nam='PedalTrack1'  show_more=off  name_source=Use Parameter  read_level=1  view_as=Number  enum_struct={'Disabled', 'Enabled'}  vector_style=Wide Row  use_help_units=off  help=''  units=''  use_header_enum=off  row_header_enum={}  col_header_enum={}  use_min_max=off  min_val=-inf  max_val=inf  use_precision=off  precision=''  gain=1  offset=0  exp=1  use_mototune_group=off  mototune_group=motohawk_vardec_path(gcb)
  motohawk_probe1 : MotoHawk_lib/Calibration & Probing Blocks/motohawk_probe  nam='PedalTrack2'  show_more=off  name_source=Use Parameter  read_level=1  view_as=Number  enum_struct={'Disabled', 'Enabled'}  vector_style=Wide Row  use_help_units=off  help=''  units=''  use_header_enum=off  row_header_enum={}  col_header_enum={}  use_min_max=off  min_val=-inf  max_val=inf  use_precision=off  precision=''  gain=1  offset=0  exp=1  use_mototune_group=off  mototune_group=motohawk_vardec_path(gcb)
  motohawk_probe2 : MotoHawk_lib/Calibration & Probing Blocks/motohawk_probe  nam='PedalTrack1_Perc'  show_more=off  name_source=Use Parameter  read_level=1  view_as=Number  enum_struct={'Disabled', 'Enabled'}  vector_style=Wide Row  use_help_units=off  help=''  units=''  use_header_enum=off  row_header_enum={}  col_header_enum={}  use_min_max=off  min_val=-inf  max_val=inf  use_precision=off  precision=''  gain=1  offset=0  exp=1  use_mototune_group=off  mototune_group=motohawk_vardec_path(gcb)
  motohawk_probe3 : MotoHawk_lib/Calibration & Probing Blocks/motohawk_probe  nam='PedalTrack2_Perc'  show_more=off  name_source=Use Parameter  read_level=1  view_as=Number  enum_struct={'Disabled', 'Enabled'}  vector_style=Wide Row  use_help_units=off  help=''  units=''  use_header_enum=off  row_header_enum={}  col_header_enum={}  use_min_max=off  min_val=-inf  max_val=inf  use_precision=off  precision=''  gain=1  offset=0  exp=1  use_mototune_group=off  mototune_group=motohawk_vardec_path(gcb)
  motohawk_probe4 : MotoHawk_lib/Calibration & Probing Blocks/motohawk_probe  nam='Pedal_Percent'  show_more=off  name_source=Use Parameter  read_level=1  view_as=Number  enum_struct={'Disabled', 'Enabled'}  vector_style=Wide Row  use_help_units=off  help=''  units=''  use_header_enum=off  row_header_enum={}  col_header_enum={}  use_min_max=off  min_val=-inf  max_val=inf  use_precision=off  precision=''  gain=1  offset=0  exp=1  use_mototune_group=off  mototune_group=motohawk_vardec_path(gcb)
  ThrottlePerc : Outport
  NoErr : Outport  Port=2
  wires:
  Pot->%/1 -> ThrottlePerc/1, motohawk_probe4/1
  Pedal1/1 -> Gain/1, motohawk_probe/1
  Supply/1 -> Gain2/1
  Pedal2/1 -> Gain1/1, motohawk_probe1/1
  Gain/1 -> Divide/1
  Gain1/1 -> Divide1/2
  Gain2/1 -> Divide/2, Divide1/1
  Divide1/1 -> Gain3/1, Interval Test/1, motohawk_probe3/1
  Divide/1 -> Switch/1, Relational Operator/1, Interval Test1/1, motohawk_probe2/1
  Gain3/1 -> Switch/3, Relational Operator/2
  Relational Operator/1 -> Switch/2
  Switch/1 -> Product/2
  Interval Test1/1 -> Product/1, Logical Operator/1
  Interval Test/1 -> Product/3, Logical Operator/2
  Product/1 -> Pot->%/1
  Logical Operator/1 -> NoErr/1

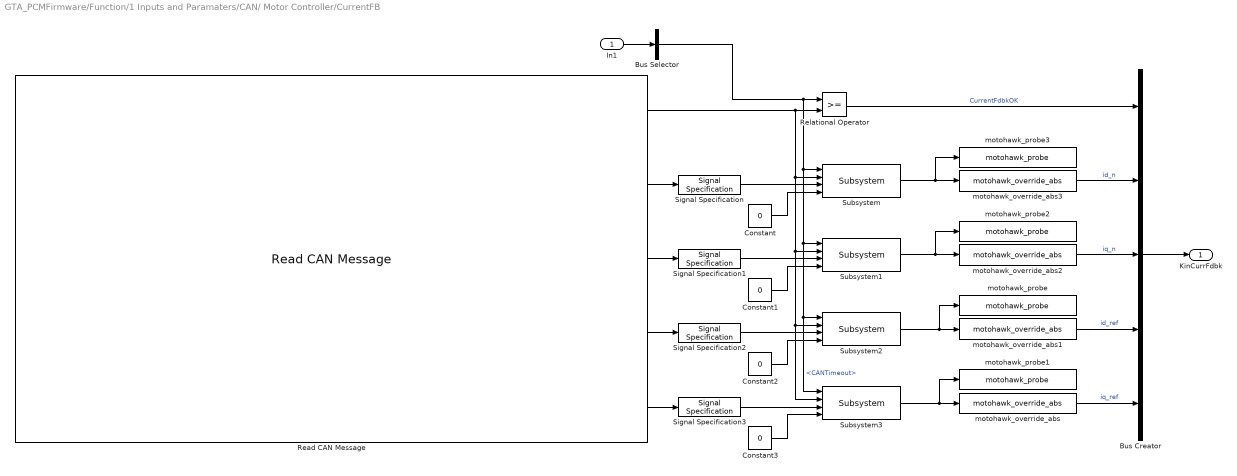
== system GTA_PCMFirmware/Function/1 Inputs and Paramaters/CAN/ Motor Controller/CurrentFB ==
  In1 : Inport
  Bus Creator : BusCreator  Inputs=5
  Bus Selector : BusSelector  OutputSignals=CANTimeout
  Constant{,1..3} (4 alike) : Constant  Value=0  OutDataTypeStr=single
  Read CAN Message : MotoHawk_lib/CAN Blocks/Read CAN Message  nam='Isolated_CAN'  bus=-2  msg=CANMSG_MCCurrentFB  queue=1  slot=''  valid=off  stale=on  labelwires=off
  Relational Operator : RelationalOperator  OutDataTypeStr=boolean
  Signal Specification{,1..3} (4 alike) : SignalSpecification  OutDataTypeStr=single
  Subsystem{,1..3} (4 alike) : GTA_Library/Subsystem
  motohawk_override_abs : MotoHawk_lib/Calibration & Probing Blocks/motohawk_override_abs  parent_name='iq_ref'  parent_val=0  show_more=off  name_source=Use Parameter  parent_read_level=1  parent_override_level=1  view_as=Number  enum_struct={'Disabled', 'Enabled'}  use_help_units=off  parent_help=''  parent_units=''  use_min_max=off  parent_min=-inf  parent_max=inf  use_precision=off  parent_precision=''  parent_gain=1  parent_offset=0  parent_exp=1  use_mototune_group=off  parent_group=motohawk_vardec_path(gcb)
  motohawk_override_abs1 : MotoHawk_lib/Calibration & Probing Blocks/motohawk_override_abs  parent_name='id_ref'  parent_val=0  show_more=off  name_source=Use Parameter  parent_read_level=1  parent_override_level=1  view_as=Number  enum_struct={'Disabled', 'Enabled'}  use_help_units=off  parent_help=''  parent_units=''  use_min_max=off  parent_min=-inf  parent_max=inf  use_precision=off  parent_precision=''  parent_gain=1  parent_offset=0  parent_exp=1  use_mototune_group=off  parent_group=motohawk_vardec_path(gcb)
  motohawk_override_abs2 : MotoHawk_lib/Calibration & Probing Blocks/motohawk_override_abs  parent_name='iq_n'  parent_val=0  show_more=off  name_source=Use Parameter  parent_read_level=1  parent_override_level=1  view_as=Number  enum_struct={'Disabled', 'Enabled'}  use_help_units=off  parent_help=''  parent_units=''  use_min_max=off  parent_min=-inf  parent_max=inf  use_precision=off  parent_precision=''  parent_gain=1  parent_offset=0  parent_exp=1  use_mototune_group=off  parent_group=motohawk_vardec_path(gcb)
  motohawk_override_abs3 : MotoHawk_lib/Calibration & Probing Blocks/motohawk_override_abs  parent_name='id_n'  parent_val=0  show_more=off  name_source=Use Parameter  parent_read_level=1  parent_override_level=1  view_as=Number  enum_struct={'Disabled', 'Enabled'}  use_help_units=off  parent_help=''  parent_units=''  use_min_max=off  parent_min=-inf  parent_max=inf  use_precision=off  parent_precision=''  parent_gain=1  parent_offset=0  parent_exp=1  use_mototune_group=off  parent_group=motohawk_vardec_path(gcb)
  motohawk_probe : MotoHawk_lib/Calibration & Probing Blocks/motohawk_probe  nam='id_ref'  show_more=off  name_source=Use Parameter  read_level=1  view_as=Number  enum_struct={'Disabled', 'Enabled'}  vector_style=Wide Row  use_help_units=off  help=''  units=''  use_header_enum=off  row_header_enum={}  col_header_enum={}  use_min_max=off  min_val=-inf  max_val=inf  use_precision=off  precision=''  gain=1  offset=0  exp=1  use_mototune_group=off  mototune_group=motohawk_vardec_path(gcb)
  motohawk_probe1 : MotoHawk_lib/Calibration & Probing Blocks/motohawk_probe  nam='iq_ref'  show_more=off  name_source=Use Parameter  read_level=1  view_as=Number  enum_struct={'Disabled', 'Enabled'}  vector_style=Wide Row  use_help_units=off  help=''  units=''  use_header_enum=off  row_header_enum={}  col_header_enum={}  use_min_max=off  min_val=-inf  max_val=inf  use_precision=off  precision=''  gain=1  offset=0  exp=1  use_mototune_group=off  mototune_group=motohawk_vardec_path(gcb)
  motohawk_probe2 : MotoHawk_lib/Calibration & Probing Blocks/motohawk_probe  nam='iq_n'  show_more=off  name_source=Use Parameter  read_level=1  view_as=Number  enum_struct={'Disabled', 'Enabled'}  vector_style=Wide Row  use_help_units=off  help=''  units=''  use_header_enum=off  row_header_enum={}  col_header_enum={}  use_min_max=off  min_val=-inf  max_val=inf  use_precision=off  precision=''  gain=1  offset=0  exp=1  use_mototune_group=off  mototune_group=motohawk_vardec_path(gcb)
  motohawk_probe3 : MotoHawk_lib/Calibration & Probing Blocks/motohawk_probe  nam='id_n'  show_more=off  name_source=Use Parameter  read_level=1  view_as=Number  enum_struct={'Disabled', 'Enabled'}  vector_style=Wide Row  use_help_units=off  help=''  units=''  use_header_enum=off  row_header_enum={}  col_header_enum={}  use_min_max=off  min_val=-inf  max_val=inf  use_precision=off  precision=''  gain=1  offset=0  exp=1  use_mototune_group=off  mototune_group=motohawk_vardec_path(gcb)
  KinCurrFdbk : Outport
  wires:
  In1/1 -> Bus Selector/1
  Read CAN Message/1 -> Relational Operator/2, Subsystem/2, Subsystem1/2, Subsystem2/2, Subsystem3/2
  Bus Selector/1 -> Relational Operator/1, Subsystem/1, Subsystem1/1, Subsystem2/1, Subsystem3/1  "<CANTimeout>"
  Read CAN Message/5 -> Signal Specification3/1
  Read CAN Message/4 -> Signal Specification2/1
  Read CAN Message/3 -> Signal Specification1/1
  Read CAN Message/2 -> Signal Specification/1
  Signal Specification/1 -> Subsystem/3
  Signal Specification3/1 -> Subsystem3/3
  Signal Specification2/1 -> Subsystem2/3
  Signal Specification1/1 -> Subsystem1/3
  Constant/1 -> Subsystem/4
  Constant1/1 -> Subsystem1/4
  Constant2/1 -> Subsystem2/4
  Constant3/1 -> Subsystem3/4
  Subsystem3/1 -> motohawk_override_abs/1, motohawk_probe1/1
  Subsystem/1 -> motohawk_override_abs3/1, motohawk_probe3/1
  Subsystem1/1 -> motohawk_override_abs2/1, motohawk_probe2/1
  Subsystem2/1 -> motohawk_override_abs1/1, motohawk_probe/1
  Relational Operator/1 -> Bus Creator/1  "CurrentFdbkOK"
  motohawk_override_abs/1 -> Bus Creator/5  "iq_ref"
  motohawk_override_abs1/1 -> Bus Creator/4  "id_ref"
  motohawk_override_abs2/1 -> Bus Creator/3  "iq_n"
  motohawk_override_abs3/1 -> Bus Creator/2  "id_n"
  Bus Creator/1 -> KinCurrFdbk/1
